simulink model "putt"  (Simulink 8.5)
settings: Solver=ode45  SolverMode=SingleTasking  StartTime=0.0  StopTime=6  MaxStep=.002  RelTol=1e-3  AbsTol=1e-6
settings Model: Creator=PC  LastModifiedBy=PC  ExtModeTrigMode=oneshot  ExtModeArmWhenConnect=off
settings DataIOCC: LimitDataPoints=off
settings OptimizationCC: BlockReduction=off  BooleanDataType=off  ExpressionDepthLimit=128
settings DebuggingCC: SaveWithParameterizedLinksMsg=none  SignalResolutionControl=TryResolveAllWithWarning  MultiTaskDSMMsg=warning  MultiTaskCondExecSysMsg=none  FcnCallInpInsideContextMsg=EnableAllAsError  StateNameClashWarn=none
settings HardwareCC: TargetUnknown=on

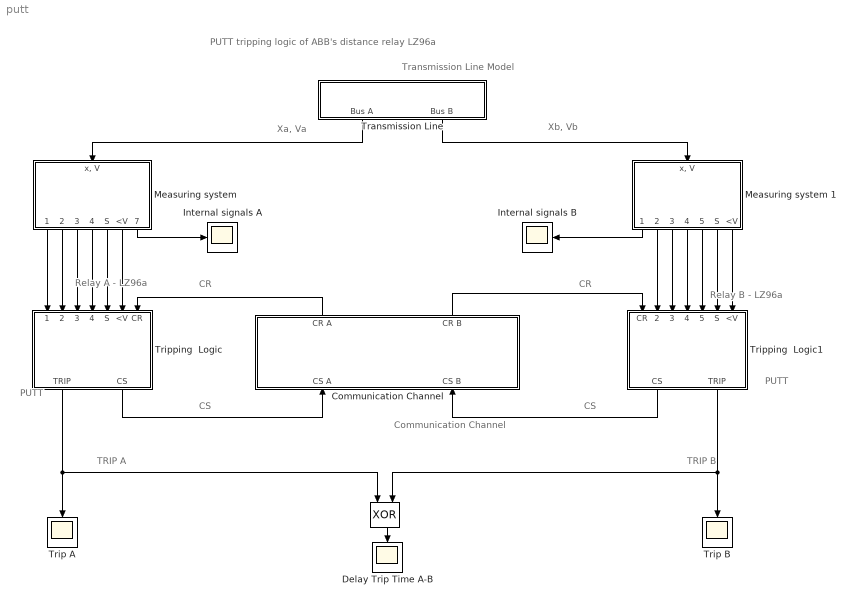
== system putt ==
  note: Transmission Line Model
  note: Relay A - LZ96a
  note: Xa, Va
  note: Xb, Vb
  note: CS
  note: CS
  note: CR
  note: CR
  note: TRIP A
  note: TRIP B
  note: PUTT tripping logic of ABB's distance relay LZ96a
  note: Relay B - LZ96a
  note: PUTT
  note: PUTT
  note: Communication
      | Channel
  " " : Logic  Operator=XOR
  Communication Channel : Subsystem  mask(Communication channel.){Tdelay=0, failureA=on, failureB=on, err_signal=0}
      mask prompts: Tdelay "Channel delay time [ms]:"; failureA "A to B Communication channel failure."; failureB "B to A Communication Channel failure"; err_signal "Erroneous signal:"
      mask TypeOptions err_signal: 0 | 1
  Delay Trip Time A-B : Scope
      settings: TickLabels=on  YMin=-0.5  YMax=2
  Internal signals A : Scope
      settings: TickLabels=on  YMin=-1  YMax=7
  Internal signals B : Scope
      settings: TickLabels=on  YMin=-1  YMax=7
  Measuring system : Subsystem  mask(Measuring system - starter block){ZM=[0.75 1.3 1.8], Tzone=[0 1 2], S=[-1 4], Tstarter=4, Vmin=0.80}
      mask prompts: ZM "Zone reach [z1 z2  z3]  [p.u.]:"; Tzone "Zone times [z1 z2  z3]  [s]:"; S "Starter range [Smin Smax] [p.u.]:"; Tstarter "Starter time [s]:"; Vmin "Undervoltage threshold V [pu.]:"
  Measuring system 1 : Subsystem  mask(Measuring system - starter block){ZM=[0.75 1.3 1.8], Tzone=[0 1 2], S=[-1 4], Tstarter=4, Vmin=0.80}
      mask prompts: ZM "Zone reach [z1 z2  z3]  [p.u.]:"; Tzone "Zone times [z1 z2  z3]  [s]:"; S "Starter range [Smin Smax] [p.u.]:"; Tstarter "Starter time [s]:"; Vmin "Undervoltage threshold V [pu.]:"
  Transmission Line : Subsystem  mask(Model of transmission line with fault){x=0.3, Tfault=0.5, Vfault=[0.90 0.75]}
      mask prompts: x "Fault location from bus A [p.u.]"; Tfault "Fault time [s]:"; Vfault "Post-fault voltages [Va  Vb] [p.u.]:"
  Trip A : Scope
      settings: TickLabels=on  YMin=-0.5  YMax=2
  Trip B : Scope
      settings: TickLabels=on  YMin=-0.5  YMax=2
  Tripping  Logic : Subsystem  mask(Tripping Logic){}
  Tripping  Logic1 : Subsystem  mask(Tripping Logic){}
  wires:
  Transmission Line/1(Bus A) -> Measuring system/1("x, V")
  Transmission Line/2(Bus B) -> Measuring system 1/1("x, V")
  Tripping  Logic1/2(TRIP) -> Trip B/1, " "/2
  Tripping  Logic/1(TRIP) -> Trip A/1, " "/1
  Measuring system/1(ZM1*t1) -> Tripping  Logic/1(ZM1*t1)
  Measuring system/2(ZM2*t2) -> Tripping  Logic/2(ZM2*t2)
  Measuring system/3(ZM3*t3) -> Tripping  Logic/3(ZM3*t3)
  Measuring system/4(S*t4) -> Tripping  Logic/4(S*t4)
  Measuring system/5(S) -> Tripping  Logic/5(S)
  Measuring system/6(<V) -> Tripping  Logic/6(<V)
  Measuring system/7(inter. signals) -> Internal signals A/1
  Measuring system 1/7(<V) -> Tripping  Logic1/7(<V)
  Measuring system 1/6(S) -> Tripping  Logic1/6(S)
  Measuring system 1/5(S*t4) -> Tripping  Logic1/5(S*t4)
  Measuring system 1/4(ZM3*t3) -> Tripping  Logic1/4(ZM3*t3)
  Measuring system 1/3(ZM2*t2) -> Tripping  Logic1/3(ZM2*t2)
  Measuring system 1/2(ZM1*t1) -> Tripping  Logic1/2(ZM1*t1)
  Measuring system 1/1(inter. signals) -> Internal signals B/1
  " "/1 -> Delay Trip Time A-B/1
  Tripping  Logic1/1(CS) -> Communication Channel/2(CS B)
  Tripping  Logic/2(CS) -> Communication Channel/1(CS A)
  Communication Channel/1(CR A) -> Tripping  Logic/7(CR)
  Communication Channel/2(CR B) -> Tripping  Logic1/1(CR)

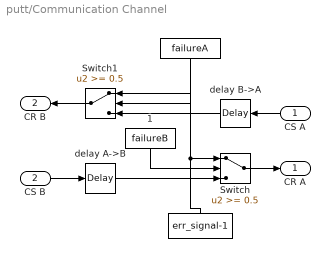
== system putt/Communication Channel ==
  CS A : Inport
  CS B : Inport  Port=2
  " " : Constant  Value=failureA
  "  " : Constant  Value=err_signal-1
  " 1" : Constant  Value=failureB
  Switch : Switch  Threshold=0.5  SaturateOnIntegerOverflow=on  InputSameDT=on
  Switch1 : Switch  Threshold=0.5  SaturateOnIntegerOverflow=on  InputSameDT=on
  delay A->B : TransportDelay  DelayTime=Tdelay/1000+1e-12
  delay B->A : TransportDelay  DelayTime=Tdelay/1000+1e-12
  CR A : Outport  InitialOutput=0
  CR B : Outport  Port=2  InitialOutput=0
  wires:
  Switch/1 -> CR A/1
  CS B/1 -> delay A->B/1
  CS A/1 -> delay B->A/1
  Switch1/1 -> CR B/1
  "  "/1 -> Switch1/1, Switch/1
  delay A->B/1 -> Switch/3
  delay B->A/1 -> Switch1/3
  " "/1 -> Switch1/2
  " 1"/1 -> Switch/2

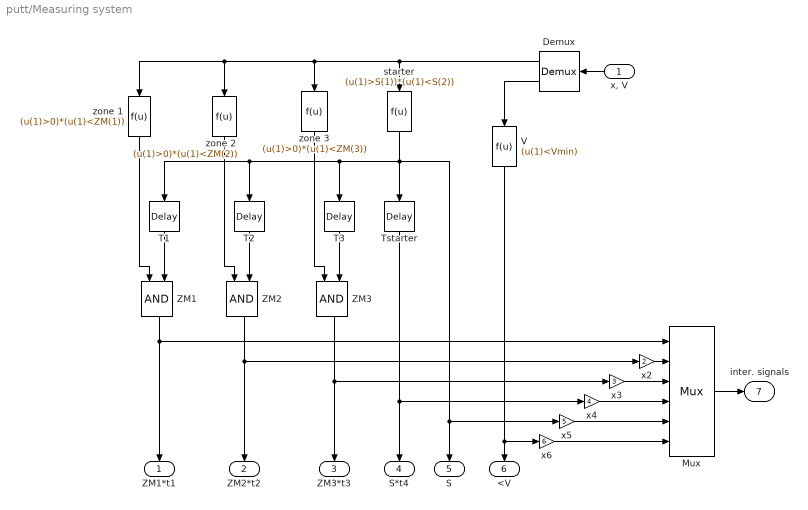
== system putt/Measuring system ==
  "x, V" : Inport
  " T1" : TransportDelay  DelayTime=Tzone(1)+1e-12
  " T2" : TransportDelay  DelayTime=Tzone(2)
  " T3" : TransportDelay  DelayTime=Tzone(3)
  " Tstarter" : TransportDelay  DelayTime=Tstarter  BufferSize=2048
  " ZM1" : Logic
  " ZM2" : Logic
  " ZM3" : Logic
  Demux : Demux  Outputs=2
  Mux : Mux  Inputs=6
  V : Fcn  Expr=(u(1)<Vmin)
  starter : Fcn  Expr=(u(1)>S(1))*(u(1)<S(2))
  x2 : Gain  Gain=2  SaturateOnIntegerOverflow=on  OutDataTypeStr=Inherit: Same as input  ParamDataTypeStr=Inherit: Same as input
  x3 : Gain  Gain=3  SaturateOnIntegerOverflow=on  OutDataTypeStr=Inherit: Same as input  ParamDataTypeStr=Inherit: Same as input
  x4 : Gain  Gain=4  SaturateOnIntegerOverflow=on  OutDataTypeStr=Inherit: Same as input  ParamDataTypeStr=Inherit: Same as input
  x5 : Gain  Gain=5  SaturateOnIntegerOverflow=on  OutDataTypeStr=Inherit: Same as input  ParamDataTypeStr=Inherit: Same as input
  x6 : Gain  Gain=6  SaturateOnIntegerOverflow=on  OutDataTypeStr=Inherit: Same as input  ParamDataTypeStr=Inherit: Same as input
  zone 1 : Fcn  Expr=(u(1)>0)*(u(1)<ZM(1))
  zone 2 : Fcn  Expr=(u(1)>0)*(u(1)<ZM(2))
  zone 3 : Fcn  Expr=(u(1)>0)*(u(1)<ZM(3))
  ZM1*t1 : Outport  InitialOutput=0
  ZM2*t2 : Outport  Port=2  InitialOutput=0
  ZM3*t3 : Outport  Port=3  InitialOutput=0
  S*t4 : Outport  Port=4  InitialOutput=0
  S : Outport  Port=5  InitialOutput=0
  <V : Outport  Port=6  InitialOutput=0
  inter. signals : Outport  Port=7  InitialOutput=0
  wires:
  starter/1 -> " T2"/1, " T1"/1, " T3"/1, " Tstarter"/1, S/1, x5/1
  " T3"/1 -> " ZM3"/2
  " T2"/1 -> " ZM2"/2
  " T1"/1 -> " ZM1"/2
  zone 3/1 -> " ZM3"/1
  zone 2/1 -> " ZM2"/1
  zone 1/1 -> " ZM1"/1
  "x, V"/1 -> Demux/1
  Demux/2 -> V/1
  Demux/1 -> zone 1/1, zone 2/1, zone 3/1, starter/1
  V/1 -> <V/1, x6/1
  " Tstarter"/1 -> S*t4/1, x4/1
  " ZM3"/1 -> ZM3*t3/1, x3/1
  " ZM2"/1 -> ZM2*t2/1, x2/1
  x3/1 -> Mux/3
  x4/1 -> Mux/4
  x5/1 -> Mux/5
  x6/1 -> Mux/6
  x2/1 -> Mux/2
  " ZM1"/1 -> ZM1*t1/1, Mux/1
  Mux/1 -> inter. signals/1

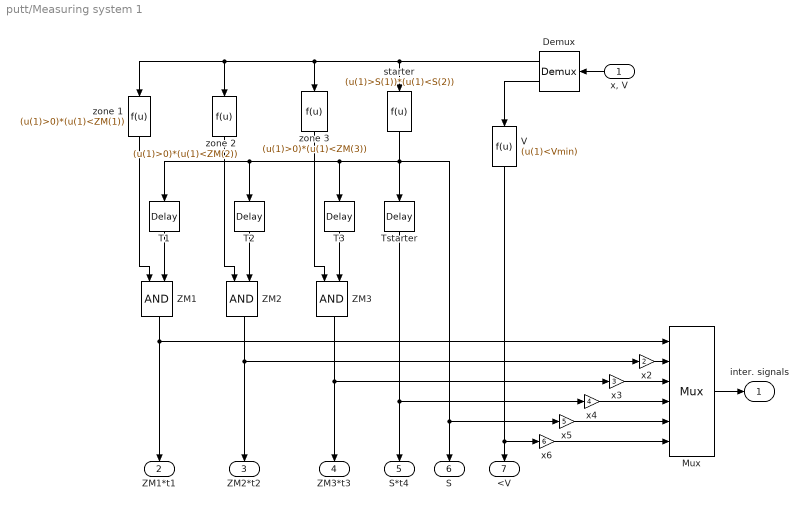
== system putt/Measuring system 1 ==
  "x, V" : Inport
  " T1" : TransportDelay  DelayTime=Tzone(1)+1e-12
  " T2" : TransportDelay  DelayTime=Tzone(2)
  " T3" : TransportDelay  DelayTime=Tzone(3)
  " Tstarter" : TransportDelay  DelayTime=Tstarter  BufferSize=2048
  " ZM1" : Logic
  " ZM2" : Logic
  " ZM3" : Logic
  Demux : Demux  Outputs=2
  Mux : Mux  Inputs=6
  V : Fcn  Expr=(u(1)<Vmin)
  starter : Fcn  Expr=(u(1)>S(1))*(u(1)<S(2))
  x2 : Gain  Gain=2  SaturateOnIntegerOverflow=on  OutDataTypeStr=Inherit: Same as input  ParamDataTypeStr=Inherit: Same as input
  x3 : Gain  Gain=3  SaturateOnIntegerOverflow=on  OutDataTypeStr=Inherit: Same as input  ParamDataTypeStr=Inherit: Same as input
  x4 : Gain  Gain=4  SaturateOnIntegerOverflow=on  OutDataTypeStr=Inherit: Same as input  ParamDataTypeStr=Inherit: Same as input
  x5 : Gain  Gain=5  SaturateOnIntegerOverflow=on  OutDataTypeStr=Inherit: Same as input  ParamDataTypeStr=Inherit: Same as input
  x6 : Gain  Gain=6  SaturateOnIntegerOverflow=on  OutDataTypeStr=Inherit: Same as input  ParamDataTypeStr=Inherit: Same as input
  zone 1 : Fcn  Expr=(u(1)>0)*(u(1)<ZM(1))
  zone 2 : Fcn  Expr=(u(1)>0)*(u(1)<ZM(2))
  zone 3 : Fcn  Expr=(u(1)>0)*(u(1)<ZM(3))
  inter. signals : Outport  InitialOutput=0
  ZM1*t1 : Outport  Port=2  InitialOutput=0
  ZM2*t2 : Outport  Port=3  InitialOutput=0
  ZM3*t3 : Outport  Port=4  InitialOutput=0
  S*t4 : Outport  Port=5  InitialOutput=0
  S : Outport  Port=6  InitialOutput=0
  <V : Outport  Port=7  InitialOutput=0
  wires:
  Mux/1 -> inter. signals/1
  " ZM1"/1 -> Mux/1, ZM1*t1/1
  x2/1 -> Mux/2
  x6/1 -> Mux/6
  x5/1 -> Mux/5
  x4/1 -> Mux/4
  x3/1 -> Mux/3
  " ZM2"/1 -> x2/1, ZM2*t2/1
  " ZM3"/1 -> x3/1, ZM3*t3/1
  " Tstarter"/1 -> x4/1, S*t4/1
  V/1 -> x6/1, <V/1
  Demux/1 -> starter/1, zone 3/1, zone 2/1, zone 1/1
  Demux/2 -> V/1
  "x, V"/1 -> Demux/1
  zone 1/1 -> " ZM1"/1
  zone 2/1 -> " ZM2"/1
  zone 3/1 -> " ZM3"/1
  " T1"/1 -> " ZM1"/2
  " T2"/1 -> " ZM2"/2
  " T3"/1 -> " ZM3"/2
  starter/1 -> x5/1, S/1, " Tstarter"/1, " T3"/1, " T1"/1, " T2"/1

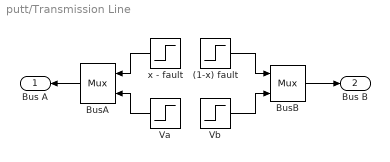
== system putt/Transmission Line ==
  (1-x) fault : Step  Time=Tfault  Before=1000  After=1-x  SampleTime=0
  BusA : Mux  Inputs=2
  BusB : Mux  Inputs=2
  Va : Step  Time=Tfault  Before=1.05  After=Vfault(1)  SampleTime=0
  Vb : Step  Time=Tfault  Before=1.05  After=Vfault(2)  SampleTime=0
  x - fault : Step  Time=Tfault  Before=1000  After=x  SampleTime=0
  Bus A : Outport  InitialOutput=0
  Bus B : Outport  Port=2  InitialOutput=0
  wires:
  Vb/1 -> BusB/2
  Va/1 -> BusA/2
  x - fault/1 -> BusA/1
  BusA/1 -> Bus A/1
  (1-x) fault/1 -> BusB/1
  BusB/1 -> Bus B/1

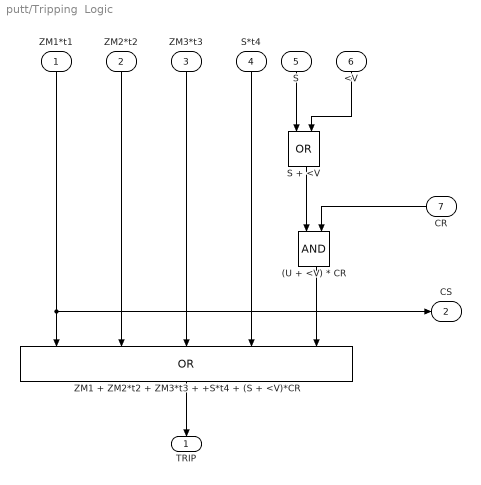
== system putt/Tripping  Logic ==
  ZM1*t1 : Inport
  ZM2*t2 : Inport  Port=2
  ZM3*t3 : Inport  Port=3
  S*t4 : Inport  Port=4
  S : Inport  Port=5
  <V : Inport  Port=6
  CR : Inport  Port=7
  (U + <V) * CR : Logic
  S + <V : Logic  Operator=OR
  ZM1 + ZM2*t2 + ZM3*t3 + +S*t4 + (S + <V)*CR : Logic  Operator=OR  Inputs=5
  TRIP : Outport  InitialOutput=0
  CS : Outport  Port=2  InitialOutput=0
  wires:
  (U + <V) * CR/1 -> ZM1 + ZM2*t2 + ZM3*t3 + +S*t4 + (S + <V)*CR/5
  ZM1 + ZM2*t2 + ZM3*t3 + +S*t4 + (S + <V)*CR/1 -> TRIP/1
  ZM2*t2/1 -> ZM1 + ZM2*t2 + ZM3*t3 + +S*t4 + (S + <V)*CR/2
  ZM3*t3/1 -> ZM1 + ZM2*t2 + ZM3*t3 + +S*t4 + (S + <V)*CR/3
  S*t4/1 -> ZM1 + ZM2*t2 + ZM3*t3 + +S*t4 + (S + <V)*CR/4
  S/1 -> S + <V/1
  <V/1 -> S + <V/2
  S + <V/1 -> (U + <V) * CR/1
  CR/1 -> (U + <V) * CR/2
  ZM1*t1/1 -> ZM1 + ZM2*t2 + ZM3*t3 + +S*t4 + (S + <V)*CR/1, CS/1

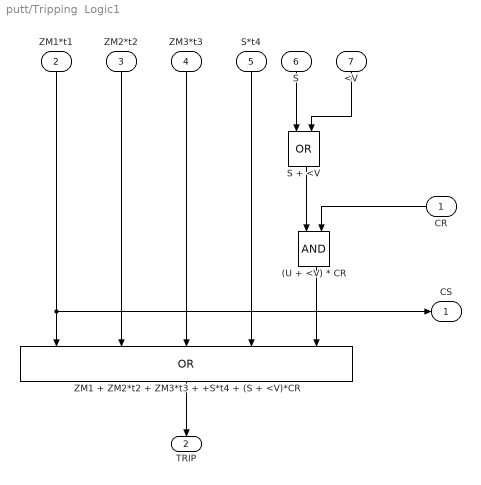
== system putt/Tripping  Logic1 ==
  CR : Inport
  ZM1*t1 : Inport  Port=2
  ZM2*t2 : Inport  Port=3
  ZM3*t3 : Inport  Port=4
  S*t4 : Inport  Port=5
  S : Inport  Port=6
  <V : Inport  Port=7
  (U + <V) * CR : Logic
  S + <V : Logic  Operator=OR
  ZM1 + ZM2*t2 + ZM3*t3 + +S*t4 + (S + <V)*CR : Logic  Operator=OR  Inputs=5
  CS : Outport  InitialOutput=0
  TRIP : Outport  Port=2  InitialOutput=0
  wires:
  ZM1*t1/1 -> CS/1, ZM1 + ZM2*t2 + ZM3*t3 + +S*t4 + (S + <V)*CR/1
  CR/1 -> (U + <V) * CR/2
  S + <V/1 -> (U + <V) * CR/1
  <V/1 -> S + <V/2
  S/1 -> S + <V/1
  S*t4/1 -> ZM1 + ZM2*t2 + ZM3*t3 + +S*t4 + (S + <V)*CR/4
  ZM3*t3/1 -> ZM1 + ZM2*t2 + ZM3*t3 + +S*t4 + (S + <V)*CR/3
  ZM2*t2/1 -> ZM1 + ZM2*t2 + ZM3*t3 + +S*t4 + (S + <V)*CR/2
  ZM1 + ZM2*t2 + ZM3*t3 + +S*t4 + (S + <V)*CR/1 -> TRIP/1
  (U + <V) * CR/1 -> ZM1 + ZM2*t2 + ZM3*t3 + +S*t4 + (S + <V)*CR/5
